simulink model "BoundedTorqueControl"  (Simulink 8.6)
settings: Solver=VariableStepAuto  StartTime=0.0  StopTime=simulationTime  RelTol=1e-3
InitFcn:
  | init_BoundedTorqueControl;
undefined symbols (not defined in the file or in its folder): constraints, DiscIntNeverNeededParam, model, ROBOT_DOF, Ts
libraries: WBToolboxLibrary x16
settings Model: Creator=marie  LastModifiedBy=DanielePucci
settings DataIOCC: SaveFormat=Dataset  SignalLoggingSaveFormat=Dataset
settings OptimizationCC: ExpressionDepthLimit=128
settings DebuggingCC: UnderspecifiedInitializationDetection=Simplified  MergeDetectMultiDrivingBlocksExec=error  SolverPrmCheckMsg=none  FcnCallInpInsideContextMsg=EnableAllAsError  StateNameClashWarn=none
settings HardwareCC: ProdBitPerPointer=64  ProdLargestAtomicFloat=Float  ProdIntDivRoundTo=Zero  ProdEndianess=LittleEndian  ProdWordSize=64  ProdHWDeviceType=Intel->x86-64 (Windows64)
settings GRTTargetCC: GeneratePreprocessorConditionals=Use local settings  CombineOutputUpdateFcns=on  GRTInterface=off
settings ConfigComp: CovModelRefEnable=off

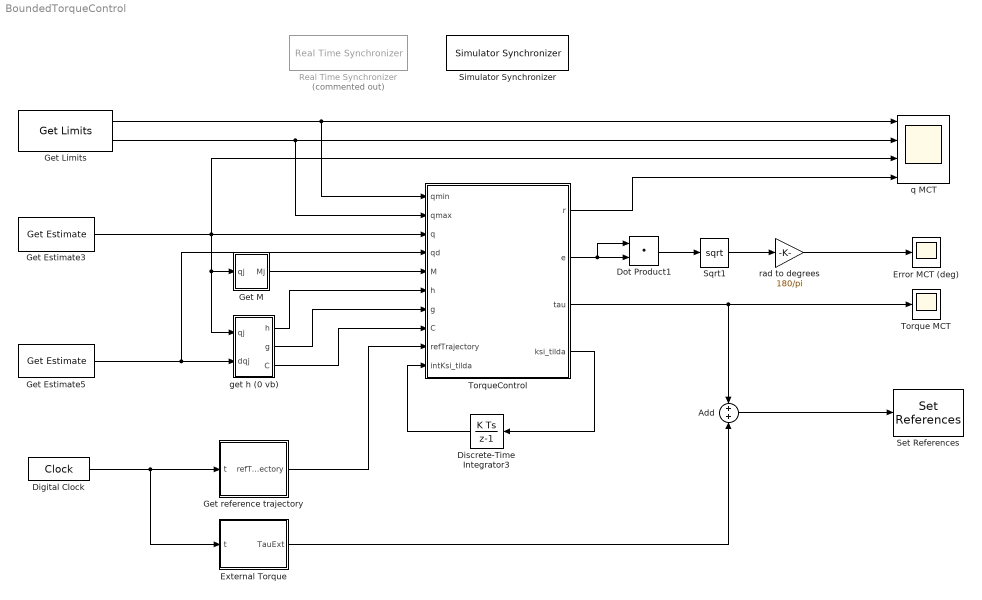
== system BoundedTorqueControl ==
  Add : Sum
  Digital Clock : DigitalClock  SampleTime=Ts
  Discrete-Time Integrator3 : DiscreteIntegrator  InitialCondition=zeros(ROBOT_DOF,1)  InitialConditionSetting=State (most efficient)  SampleTime=Ts  ICPrevOutput=DiscIntNeverNeededParam  ICPrevScaledInput=DiscIntNeverNeededParam
  Dot Product1 : DotProduct  InputSameDT=on  OutDataTypeStr=Inherit: Inherit via internal rule
  Error MCT (deg) : Scope
  External Torque : MATLAB Function  TreatAsAtomicUnit=on
  Get Estimate3 : WBToolboxLibrary/wholeBodyStates/Get Estimate  estimateType=Joints Position  robotName=WBT_robotName  localName=WBT_modelName  wbiFile=WBT_wbiFilename  wbiList=WBT_wbiList
  Get Estimate5 : WBToolboxLibrary/wholeBodyStates/Get Estimate  estimateType=Joints Velocity  robotName=WBT_robotName  localName=WBT_modelName  wbiFile=WBT_wbiFilename  wbiList=WBT_wbiList
  Get Limits : WBToolboxLibrary/wholeBodyStates/Get Limits  limitsType=Position  robotName=WBT_robotName  localName=WBT_modelName  wbiFile=WBT_wbiFilename  wbiList=WBT_wbiList
  Get M : Subsystem
  Get reference trajectory : MATLAB Function  TreatAsAtomicUnit=on
  Real Time Synchronizer : WBToolboxLibrary/Utilities/Real Time Synchronizer  Commented=on  period=Ts
  Set References : WBToolboxLibrary/wholeBodyActuators/Set References  controlType=Torque  robotName=WBT_robotName  localName=WBT_modelName  wbiFile=WBT_wbiFilename  wbiList=WBT_wbiList
  Simulator Synchronizer : WBToolboxLibrary/Utilities/Simulator Synchronizer  period=Ts  serverPortName='/clock/rpc'  clientPortName='/WBT_synchronizer/rpc:o'
  Sqrt1 : Sqrt  SaturateOnIntegerOverflow=on
  Torque MCT : Scope
  TorqueControl : MATLAB Function  TreatAsAtomicUnit=on
  get h (0 vb) : Subsystem
  q MCT : Scope  NumInputPorts=4
  rad to degrees : Gain  Gain=180/pi
  wires:
  Get Estimate3/1 -> get h (0 vb)/1(qj), Get M/1(qj), q MCT/3, TorqueControl/3(q)
  Get Estimate5/1 -> TorqueControl/4(qd), get h (0 vb)/2(dqj)
  Get M/1(Mj) -> TorqueControl/5(M)
  get h (0 vb)/1(h) -> TorqueControl/6(h)
  Get Limits/2 -> TorqueControl/2(qmax), q MCT/2
  Get Limits/1 -> TorqueControl/1(qmin), q MCT/1
  TorqueControl/3(tau) -> Torque MCT/1, Add/1
  TorqueControl/4(ksi_tilda) -> Discrete-Time Integrator3/1
  Discrete-Time Integrator3/1 -> TorqueControl/10(intKsi_tilda)
  TorqueControl/2(e) -> Dot Product1/1, Dot Product1/2
  Dot Product1/1 -> Sqrt1/1
  Sqrt1/1 -> rad to degrees/1
  rad to degrees/1 -> Error MCT (deg)/1
  Add/1 -> Set References/1
  Digital Clock/1 -> External Torque/1(t), Get reference trajectory/1(t)
  External Torque/1(TauExt) -> Add/2
  Get reference trajectory/1(refTrajectory) -> TorqueControl/9(refTrajectory)
  TorqueControl/1(r) -> q MCT/4
  get h (0 vb)/2(g) -> TorqueControl/7(g)
  get h (0 vb)/3(C) -> TorqueControl/8(C)

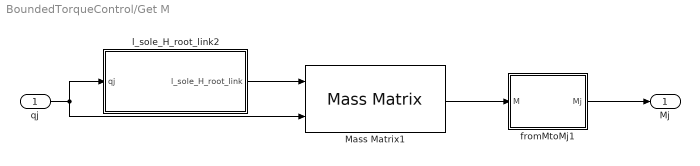
== system BoundedTorqueControl/Get M ==
  qj : Inport
  Mass Matrix1 : WBToolboxLibrary/wholeBodyModel/Dynamics/Mass Matrix  robotName=WBT_robotName  localName=WBT_modelName  wbiFile=WBT_wbiFilename  wbiList=WBT_wbiList
  fromMtoMj1 : MATLAB Function  TreatAsAtomicUnit=on
  l_sole_H_root_link2 : Subsystem
  Mj : Outport
  wires:
  fromMtoMj1/1(Mj) -> Mj/1
  qj/1 -> l_sole_H_root_link2/1(qj), Mass Matrix1/2
  Mass Matrix1/1 -> fromMtoMj1/1(M)
  l_sole_H_root_link2/1(l_sole_H_root_link) -> Mass Matrix1/1

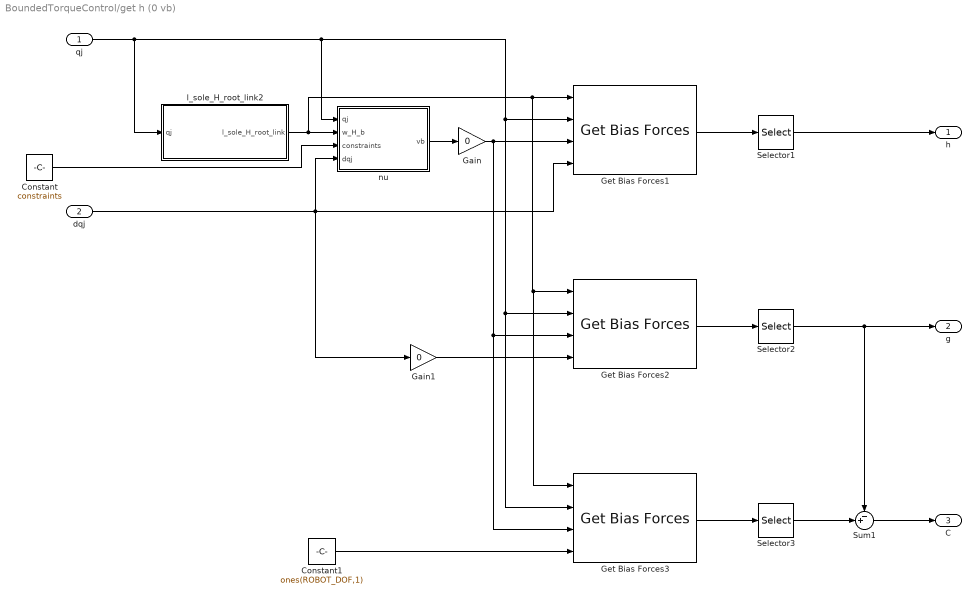
== system BoundedTorqueControl/get h (0 vb) ==
  qj : Inport
  dqj : Inport  Port=2
  Constant : Constant  Value=constraints
  Constant1 : Constant  Value=ones(ROBOT_DOF,1)
  Gain : Gain  Gain=0
  Gain1 : Gain  Gain=0
  Get Bias Forces1 : WBToolboxLibrary/wholeBodyModel/Dynamics/Get Bias Forces  robotName=WBT_robotName  localName=WBT_modelName  wbiFile=WBT_wbiFilename  wbiList=WBT_wbiList
  Get Bias Forces2 : WBToolboxLibrary/wholeBodyModel/Dynamics/Get Bias Forces  robotName=WBT_robotName  localName=WBT_modelName  wbiFile=WBT_wbiFilename  wbiList=WBT_wbiList
  Get Bias Forces3 : WBToolboxLibrary/wholeBodyModel/Dynamics/Get Bias Forces  robotName=WBT_robotName  localName=WBT_modelName  wbiFile=WBT_wbiFilename  wbiList=WBT_wbiList
  Selector1 : Selector  InputPortWidth=ROBOT_DOF+6  IndexOptions=Index vector (dialog)  Indices=[7:ROBOT_DOF+6]  OutputSizes=1
  Selector2 : Selector  InputPortWidth=ROBOT_DOF+6  IndexOptions=Index vector (dialog)  Indices=[7:ROBOT_DOF+6]  OutputSizes=1
  Selector3 : Selector  InputPortWidth=ROBOT_DOF+6  IndexOptions=Index vector (dialog)  Indices=[7:ROBOT_DOF+6]  OutputSizes=1
  Sum1 : Sum  Inputs=-+|
  l_sole_H_root_link2 : Subsystem
  nu : Subsystem
  h : Outport
  g : Outport  Port=2
  C : Outport  Port=3
  wires:
  Get Bias Forces1/1 -> Selector1/1
  qj/1 -> l_sole_H_root_link2/1(qj), Get Bias Forces3/2, Get Bias Forces2/2, Get Bias Forces1/2, nu/1(qj)
  l_sole_H_root_link2/1(l_sole_H_root_link) -> nu/2(w_H_b), Get Bias Forces3/1, Get Bias Forces2/1, Get Bias Forces1/1
  nu/1(vb) -> Gain/1
  Gain/1 -> Get Bias Forces1/3, Get Bias Forces3/3, Get Bias Forces2/3
  Constant/1 -> nu/3("constraints ")
  Gain1/1 -> Get Bias Forces2/4
  Get Bias Forces2/1 -> Selector2/1
  Selector2/1 -> Sum1/1, g/1
  dqj/1 -> nu/4(dqj), Get Bias Forces1/4, Gain1/1
  Get Bias Forces3/1 -> Selector3/1
  Selector3/1 -> Sum1/2
  Sum1/1 -> C/1
  Constant1/1 -> Get Bias Forces3/4
  Selector1/1 -> h/1

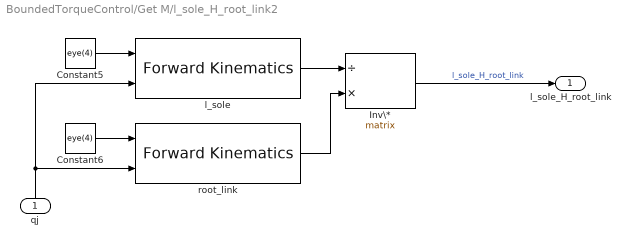
== system BoundedTorqueControl/Get M/l_sole_H_root_link2 ==
  qj : Inport
  Constant5 : Constant  Value=eye(4)
  Constant6 : Constant  Value=eye(4)
  Inv\* : Product  Inputs=/*  Multiplication=Matrix(*)
  l_sole : WBToolboxLibrary/wholeBodyModel/Kinematics/Forward Kinematics  frameName='l_sole'  robotName=WBT_robotName  localName=WBT_modelName  wbiFile=WBT_wbiFilename  wbiList=WBT_wbiList
  root_link : WBToolboxLibrary/wholeBodyModel/Kinematics/Forward Kinematics  frameName='root_link'  robotName=WBT_robotName  localName=WBT_modelName  wbiFile=WBT_wbiFilename  wbiList=WBT_wbiList
  l_sole_H_root_link : Outport
  wires:
  root_link/1 -> Inv\*/2
  qj/1 -> root_link/2, l_sole/2
  Constant6/1 -> root_link/1
  l_sole/1 -> Inv\*/1
  Inv\*/1 -> l_sole_H_root_link/1  "l_sole_H_root_link"
  Constant5/1 -> l_sole/1

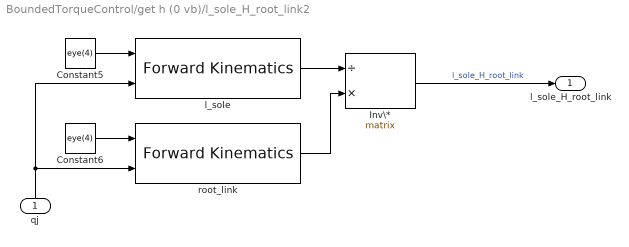
== system BoundedTorqueControl/get h (0 vb)/l_sole_H_root_link2 ==
  qj : Inport
  Constant5 : Constant  Value=eye(4)
  Constant6 : Constant  Value=eye(4)
  Inv\* : Product  Inputs=/*  Multiplication=Matrix(*)
  l_sole : WBToolboxLibrary/wholeBodyModel/Kinematics/Forward Kinematics  frameName='l_sole'  robotName=WBT_robotName  localName=WBT_modelName  wbiFile=WBT_wbiFilename  wbiList=WBT_wbiList
  root_link : WBToolboxLibrary/wholeBodyModel/Kinematics/Forward Kinematics  frameName='root_link'  robotName=WBT_robotName  localName=WBT_modelName  wbiFile=WBT_wbiFilename  wbiList=WBT_wbiList
  l_sole_H_root_link : Outport
  wires:
  root_link/1 -> Inv\*/2
  qj/1 -> root_link/2, l_sole/2
  Constant6/1 -> root_link/1
  l_sole/1 -> Inv\*/1
  Inv\*/1 -> l_sole_H_root_link/1  "l_sole_H_root_link"
  Constant5/1 -> l_sole/1

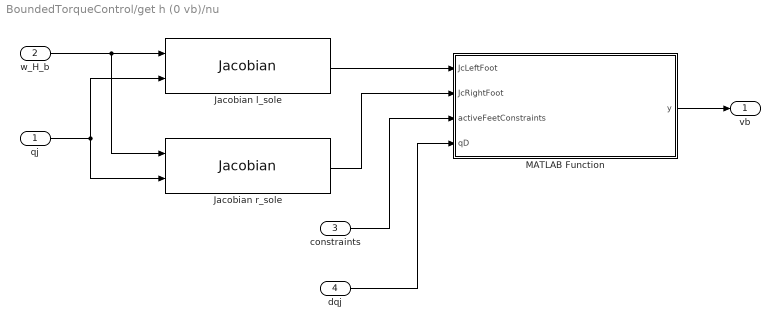
== system BoundedTorqueControl/get h (0 vb)/nu ==
  qj : Inport
  w_H_b : Inport  Port=2
  "constraints " : Inport  Port=3
  dqj : Inport  Port=4
  Jacobian l_sole : WBToolboxLibrary/wholeBodyModel/Jacobians/Jacobian  frameName='l_sole'  robotName=WBT_robotName  localName=WBT_modelName  wbiFile=WBT_wbiFilename  wbiList=WBT_wbiList
  Jacobian r_sole : WBToolboxLibrary/wholeBodyModel/Jacobians/Jacobian  frameName='r_sole'  robotName=WBT_robotName  localName=WBT_modelName  wbiFile=WBT_wbiFilename  wbiList=WBT_wbiList
  MATLAB Function : MATLAB Function  TreatAsAtomicUnit=on
  vb : Outport
  wires:
  dqj/1 -> MATLAB Function/4(qD)
  Jacobian r_sole/1 -> MATLAB Function/2(JcRightFoot)
  "constraints "/1 -> MATLAB Function/3(activeFeetConstraints)
  MATLAB Function/1(y) -> vb/1
  Jacobian l_sole/1 -> MATLAB Function/1(JcLeftFoot)
  qj/1 -> Jacobian r_sole/2, Jacobian l_sole/2
  w_H_b/1 -> Jacobian l_sole/1, Jacobian r_sole/1

== matlab function TorqueControl ==
  data: r output double; ROBOT_DOF parameter double; model parameter double; qmin input double; qmax input double; q input double; qd input double; M input double; h input double; g input double; C input double; refTrajectory input double; intKsi_tilda input double; e output double; tau output double; ksi_tilda output double
function [r, e, tau, ksi_tilda] = fcn(ROBOT_DOF, model, qmin, qmax, q, qd, M, h, g, C, refTrajectory, intKsi_tilda)

%Computed torque control

%Input:
%ROBOT_DOF: number of degrees of freedom of the robot
%model: parameter defined in the init script, containing control gains
%qmin: vector of minimum joint limits
%qmax: vector of maximum joint limits
%q: vector of joint positions
%qd: vector of joint velocities
%M: inertia matrix
%h: matrix combining gravity, coriolis and friction torques
%refTrajectory: reference joint position trajectory r, in the shape [r; rd; rdd]
    %r: position reference trajectory
    %rd: velocity reference trajectory
    %rdd: acceleration reference trajectory
%intKsi_tilda: integral of the position tracking error


%Output:
%r: position reference trajectory
%e: position tracking error
%tau: vector of input motor torques
%ksi_tilda: position tracking error in terms of parameter ksi


q0 = (qmin + qmax)/2;
delta = (qmax - qmin)/2;

r = refTrajectory(1 : ROBOT_DOF);
rd = refTrajectory(ROBOT_DOF + 1 : 2 * ROBOT_DOF);
rdd = refTrajectory(2 * ROBOT_DOF + 1 : 3 * ROBOT_DOF);
e = q - r;
ed = qd - rd;

%convert reference trajectory and state in terms of ksi
ksi = zeros(ROBOT_DOF, 1);
ksid = zeros(ROBOT_DOF, 1);
ksi_r = zeros(ROBOT_DOF, 1);
ksi_rd = zeros(ROBOT_DOF, 1);
ksi_rdd = zeros(ROBOT_DOF,1);

for i = 1:ROBOT_DOF
    ksi_r(i) = atanh((r(i) - q0(i))/delta(i));
    ksi_rd(i) = rd(i) / (delta(i) * (1 - tanh(ksi_r(i))^2));
    ksi_rdd(i) = rdd(i)/(delta(i) * (1 - tanh(ksi_r(i))^2)) + 2 * tanh(ksi_r(i)) * ksi_rd(i)^2;
    
    ksi(i) = atanh((q(i) - q0(i))/delta(i));
    ksid(i) = qd(i) / (delta(i) * (1 - tanh(ksi(i))^2));
end

% get error on ksi
ksi_tilda = ksi - ksi_r;
ksi_tildad = ksid - ksi_rd;


%% Control schemes: uncomment the one you wish to use

% %Computed torque
% ksiddstar = ksi_rdd - model.Kp * ksi_tilda - model.Kd * ksi_tildad - model.Ki * intKsi_tilda;
% tau = M * ksiddstar + h; % h = g + C * qd;

% %Gravity compensation, neglecting M*ksi_rdd and C*ksi_d
J_ksi = diag(delta .* (1 - tanh(ksi).^2));
tau = g - J_ksi\ (model.Kp * ksi_tilda + model.Kd * ksi_tildad + model.Ki * intKsi_tilda);

% %Gravity compensation, including M*ksi_rdd and C*ksi_d
% J_ksi = diag(delta .* (1 - tanh(ksi).^2));
% J_ksid = diag( - 2 * delta .* tanh(ksi) .* (1 - tanh(ksi).^2) .* ksid);
% tau = M * J_ksi * ksi_rdd + (M * J_ksid + C * J_ksi) * ksi_rd + g - J_ksi' \ model.Kp * ksi_tilda - J_ksi' \ model.Kd * ksi_tildad - J_ksi' \ model.Ki * intKsi_tilda;


%Gravity compensation, no variable change to ksi
% tau = M * rdd + C * rd + g - J_ksi' \ model.Kp * e - J_ksi' \ model.Kd * ed;

== matlab function Get reference trajectory ==
  data: refTrajectory output double; t input double; model parameter double
function refTrajectory  = fcn(t, model)
%t: simulation time
%r, rd, rdd: reference trajectory
%knee joint limits -2.1817:0.4014

switch model.trajectory
  
    case 1
        %Ramped reference trajectory towards minimum/maximum joint limit
        r = model.p * t + model.r0;
        rd = model.p;
        rdd = 0;
        if r >= model.rmax
            r = model.rmax;
            rd = 0;
        end
        if r <= model.rmin
            r = model.rmin;
            rd = 0;
        end
        
    case 2
        %Sinusoidal reference trajectory
        r = model.rAmplitude * sin(model.rFrequency * t) + model.rbias;
        rd = model.rFrequency * model.rAmplitude * cos(model.rFrequency * t);
        rdd = - model.rFrequency^2 * model.rAmplitude * sin(model.rFrequency * t);
        
    otherwise
        r = 0; rd = 0; rdd = 0;
end

refTrajectory = [r; rd; rdd];

== matlab function External Torque ==
  data: TauExt output double; t input double; model parameter double
function TauExt = fcn(t, model)
%t: simulation time

%Apply an external torque to the joint
if t >= model.TextIniTime && t <= model.TextEndTime
    TauExt = model.Text;
else
    TauExt = 0;
end

== matlab function Get M/fromMtoMj1 ==
  data: M input double; Mj output double
function Mj = fromMtoMj(M)
%#codegen

Mj = M(7:end,7:end);

== matlab function get h (0 vb)/nu/MATLAB Function ==
  data: JcLeftFoot input double; JcRightFoot input double; activeFeetConstraints input double; y output double; qD input double
function y = fcn(JcLeftFoot,JcRightFoot,activeFeetConstraints,qD)
%#codegen
reg = 1e-5;

Jc  = [activeFeetConstraints(1)*JcLeftFoot;
       activeFeetConstraints(2)*JcRightFoot];

pinvJb = (Jc(:,1:6)'*Jc(:,1:6) + reg*eye(6))\Jc(:,1:6)';  
  
% pinvJb = pinv(Jc(:,1:6));

y = -pinvJb*Jc(:,7:end)*qD;
